simulink model "eco_Simulink"  (R2020b)
settings: Solver=VariableStepAuto  StartTime=0.0  StopTime=10  RelTol=1e-3
libraries: dspsnks4 x1, dspvision x1
settings Model: Creator=JonathanPC  LastModifiedBy=JonathanPC

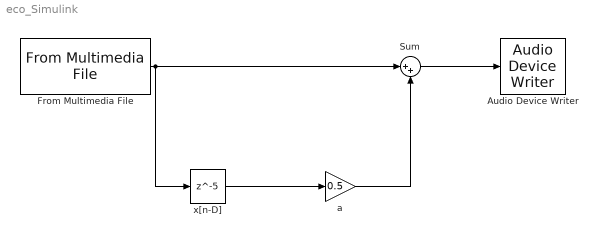
== system eco_Simulink ==
  Audio Device Writer : dspsnks4/Audio Device Writer  Driver=DirectSound  Device=Default  InheritSampleRate=on  SampleRate=44100  BitDepth=16-bit integer  BufferSize=4096  NumBuffers=10  DefaultOutputChannelMapping=on  OutputChannelMapping=1:2  OutputNumUnderrunSamples=off  DriverIdx=1  DeviceWarnFlag=''
  From Multimedia File : dspvision/From Multimedia File  inputFilename=C:\Users\JonathanPC\Documents\MATLAB\taller2\Sonido.wav  readRange=[1 Inf]  loop=on  numPlays=inf  outputStreams=Audio only  videoDataType=single  audioDataType=double  inheritSampleTime=on  userDefinedSampleTime=1/30  noAudioOutput=off  isIntensityVideo=off  fourcc=RGB  colorVideoFormat=Separate color signals  outputEOF=off  dataOrg=Column-major  audioFrameSize=1024  computeAudioFrameSize=off  outSamplingMode=Sample based
  Sum : Sum  Inputs=|++
  a : Gain  Gain=0.5
  x[n-D] : Delay  DelayLength=5
  wires:
  From Multimedia File/1 -> Sum/1, x[n-D]/1
  x[n-D]/1 -> a/1
  Sum/1 -> Audio Device Writer/1
  a/1 -> Sum/2
